simulink library "quat_rectify_lib"  (R2018b)
settings: Solver=VariableStepAuto  StartTime=0.0  StopTime=10.0  RelTol=1e-3
settings Model: Creator=Taylor  LastModifiedBy=Taylor

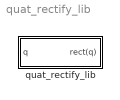
== system quat_rectify_lib ==
  quat_rectify_lib : Subsystem  TreatAsAtomicUnit=on
      settings: RTWFcnNameOpts=Use subsystem name  RTWFileNameOpts=Use subsystem name
      mask DialogControl DescGroupVar Prompt: Quaternion Rectification
      mask DialogControl DescTextVar Prompt: The quaternions output by this block always have a nonnegative scalar part.

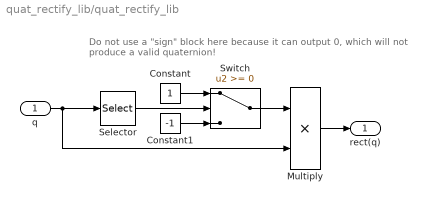
== system quat_rectify_lib/quat_rectify_lib ==
  note: Do not use a "sign" block here because it can
      | output 0, which will not produce a valid quaternion!
  q : Inport
  Constant : Constant
  Constant1 : Constant  Value=-1
  Multiply : Product
  Selector : Selector  InputPortWidth=4  IndexOptions=Index vector (dialog)  Indices=[1]  OutputSizes=1
  Switch : Switch
  rect(q) : Outport
  wires:
  q/1 -> Multiply/2, Selector/1
  Switch/1 -> Multiply/1
  Selector/1 -> Switch/2
  Multiply/1 -> rect(q)/1
  Constant/1 -> Switch/1
  Constant1/1 -> Switch/3
